simulink model "MainSimLoop"  (R2020b)
settings: Solver=VariableStepAuto  StartTime=0.0  StopTime=30  RelTol=1e-3
values from neighbouring files (symbols this model uses):
  D = 12    [Startup.m]
  dctcq = [-2.56941525e-08,-5.1388305e-08,-2.56941525e-08,2.56941525e-08,5.1388305e-08,2.56941525e-08;     4.45035775874229e-08,0,-4.45035775874229e-08,-4.45035775874229e-08,0,4.45035775874229e-08;     2.925e-09,-2.925e-09,2.925e-09,-2.925e-09,2.925e-09,-2.925e-09]    [Startup.m]
  Jm = 2.9387e-05    [Startup.m]
  mass = 3.3    [Startup.m]
  P = 3.8    [Startup.m]
  X = [ 0, 0, 5, 5, 5, 5, 0]*1    [Path_Construction_Demo_Script.m]
  Y = [ 0, 0, 0, 0, 5, 5, 5]*1    [Path_Construction_Demo_Script.m]
  Z = [ 1, 1, 1, 1, 1, 1, 1]*0    [Path_Construction_Demo_Script.m]
undefined symbols (not defined in the file or in its folder): Newton, Raphson, sigbuilder_block, smiData
libraries: sm_lib x542, fl_lib x73, nesl_utility x26, Electrical_Library x18, pid_lib x12, Mechanical_Library x12, sharedtransform x12, shared6dof x1
(part 4 of 12)

== system MainSimLoop/Quadcopter Dynamics/Motor6CCW/Subsystem ==
  ArmMotorConnector_1_RIGID : Subsystem
  ArmRod_1_RIGID : Subsystem
  LegBodyConnector_1_RIGID : Subsystem
  MotorMount_1_RIGID : Subsystem
  MotorQuad_1_RIGID : Subsystem
  Transform : sm_lib/Frames and Transforms/Rigid Transform  TranslationMethod=Cartesian  TranslationStandardOffset=0  TranslationLengthUnit=mm  TranslationStandardAxis=+Z  TranslationCartesianOffset=smiData.RigidTransform(156).translation  TranslationROffset=0  TranslationROffsetUnits=m  TranslationZOffset=0  TranslationZOffsetUnits=m  TranslationThetaOffset=0  TranslationThetaOffsetUnits=deg  RotationMethod=ArbitraryAxis  RotationAngleUnits=rad  RotationStandardAxis=+Z  RotationAngle=smiData.RigidTransform(156).angle  RotationArbitraryAxis=smiData.RigidTransform(156).axis  FollAlignAxisA=+X  BaseAlignAxisA=+Y  FollAlignAxisB=+Y  BaseAlignAxisB=+Z  RotationSequenceAxes=FollowerAxes  RotationSequence=XYX  RotationSequenceAngles=[0 0 0]  RotationSequenceAnglesUnits=deg  RotationMatrix=[1 0 0; 0 1 0; 0 0 1]
  Transform1 : sm_lib/Frames and Transforms/Rigid Transform  TranslationMethod=Cartesian  TranslationStandardOffset=0  TranslationLengthUnit=mm  TranslationStandardAxis=+Z  TranslationCartesianOffset=smiData.RigidTransform(157).translation  TranslationROffset=0  TranslationROffsetUnits=m  TranslationZOffset=0  TranslationZOffsetUnits=m  TranslationThetaOffset=0  TranslationThetaOffsetUnits=deg  RotationMethod=ArbitraryAxis  RotationAngleUnits=rad  RotationStandardAxis=+Z  RotationAngle=smiData.RigidTransform(157).angle  RotationArbitraryAxis=smiData.RigidTransform(157).axis  FollAlignAxisA=+X  BaseAlignAxisA=+Y  FollAlignAxisB=+Y  BaseAlignAxisB=+Z  RotationSequenceAxes=FollowerAxes  RotationSequence=XYX  RotationSequenceAngles=[0 0 0]  RotationSequenceAnglesUnits=deg  RotationMatrix=[1 0 0; 0 1 0; 0 0 1]
  Transform2 : sm_lib/Frames and Transforms/Rigid Transform  TranslationMethod=Cartesian  TranslationStandardOffset=0  TranslationLengthUnit=mm  TranslationStandardAxis=+Z  TranslationCartesianOffset=smiData.RigidTransform(158).translation  TranslationROffset=0  TranslationROffsetUnits=m  TranslationZOffset=0  TranslationZOffsetUnits=m  TranslationThetaOffset=0  TranslationThetaOffsetUnits=deg  RotationMethod=ArbitraryAxis  RotationAngleUnits=rad  RotationStandardAxis=+Z  RotationAngle=smiData.RigidTransform(158).angle  RotationArbitraryAxis=smiData.RigidTransform(158).axis  FollAlignAxisA=+X  BaseAlignAxisA=+Y  FollAlignAxisB=+Y  BaseAlignAxisB=+Z  RotationSequenceAxes=FollowerAxes  RotationSequence=XYX  RotationSequenceAngles=[0 0 0]  RotationSequenceAnglesUnits=deg  RotationMatrix=[1 0 0; 0 1 0; 0 0 1]
  Transform3 : sm_lib/Frames and Transforms/Rigid Transform  TranslationMethod=Cartesian  TranslationStandardOffset=0  TranslationLengthUnit=mm  TranslationStandardAxis=+Z  TranslationCartesianOffset=smiData.RigidTransform(159).translation  TranslationROffset=0  TranslationROffsetUnits=m  TranslationZOffset=0  TranslationZOffsetUnits=m  TranslationThetaOffset=0  TranslationThetaOffsetUnits=deg  RotationMethod=ArbitraryAxis  RotationAngleUnits=rad  RotationStandardAxis=+Z  RotationAngle=smiData.RigidTransform(159).angle  RotationArbitraryAxis=smiData.RigidTransform(159).axis  FollAlignAxisA=+X  BaseAlignAxisA=+Y  FollAlignAxisB=+Y  BaseAlignAxisB=+Z  RotationSequenceAxes=FollowerAxes  RotationSequence=XYX  RotationSequenceAngles=[0 0 0]  RotationSequenceAnglesUnits=deg  RotationMatrix=[1 0 0; 0 1 0; 0 0 1]
  Transform5 : sm_lib/Frames and Transforms/Rigid Transform  TranslationMethod=Cartesian  TranslationStandardOffset=0  TranslationLengthUnit=mm  TranslationStandardAxis=+Z  TranslationCartesianOffset=smiData.RigidTransform(161).translation  TranslationROffset=0  TranslationROffsetUnits=m  TranslationZOffset=0  TranslationZOffsetUnits=m  TranslationThetaOffset=0  TranslationThetaOffsetUnits=deg  RotationMethod=ArbitraryAxis  RotationAngleUnits=rad  RotationStandardAxis=+Z  RotationAngle=smiData.RigidTransform(161).angle  RotationArbitraryAxis=smiData.RigidTransform(161).axis  FollAlignAxisA=+X  BaseAlignAxisA=+Y  FollAlignAxisB=+Y  BaseAlignAxisB=+Z  RotationSequenceAxes=FollowerAxes  RotationSequence=XYX  RotationSequenceAngles=[0 0 0]  RotationSequenceAnglesUnits=deg  RotationMatrix=[1 0 0; 0 1 0; 0 0 1]
  Transform4 : PMIOPort  Side=Left
  Transform6 : PMIOPort  Port=2  Side=Left
  Transform7 : PMIOPort  Port=3  Side=Left
  connections:
  Transform6/RConn1 -- Transform3/LConn1
  Transform/LConn1 -- Transform1/LConn1 -- Transform2/LConn1 -- Transform7/RConn1
  MotorMount_1_RIGID/LConn1 -- Transform/RConn1
  Transform4/RConn1 -- Transform5/LConn1
  ArmMotorConnector_1_RIGID/LConn1 -- Transform2/RConn1
  MotorQuad_1_RIGID/LConn1 -- Transform5/RConn1
  ArmRod_1_RIGID/LConn1 -- Transform3/RConn1
  LegBodyConnector_1_RIGID/LConn1 -- Transform1/RConn1

== system MainSimLoop/Quadcopter Dynamics/Motor6CCW/xoar_12_4_5CW_1_RIGID ==
  ReferenceFrame : sm_lib/Frames and Transforms/Reference Frame
  Solid : sm_lib/Body Elements/File Solid  ExtGeomFileName=xoar_12_4-5CW_Default_sldprt.STEP  UnitType=FromFile  ExtGeomFileUnits=m  StepReaderType=HEX  ExportConvexHullGeometry=off  InertiaType=Custom  Mass=smiData.Solid(44).mass  MassUnits=kg  CenterOfMass=smiData.Solid(44).CoM  CenterOfMassUnits=m  MomentsOfInertia=smiData.Solid(44).MoI  MomentsOfInertiaUnits=kg*m^2  ProductsOfInertia=smiData.Solid(44).PoI  ProductsOfInertiaUnits=kg*m^2  BasedOnType=DensityFromFile  Density=1000  DensityUnits=kg/m^3  DoExposeReferenceFrame=on  SerializedFrames=<Frames/>  GraphicType=FromGeometry  MarkerShape=Sphere  MarkerSize=10  GraphicVisPropType=SimpleVisualProperties  GraphicDiffuseColor=smiData.Solid(44).color  GraphicSpecularColor=[0.5 0.5 0.5 1.0]  GraphicAmbientColor=[0.15 0.15 0.15 1.0]  GraphicEmissiveColor=[0.0 0.0 0.0 1.0]  GraphicShininess=75  GraphicOpacity=smiData.Solid(44).opacity
  F : PMIOPort  Side=Left
  connections:
  ReferenceFrame/RConn1 -- Solid/RConn1 -- F/RConn1

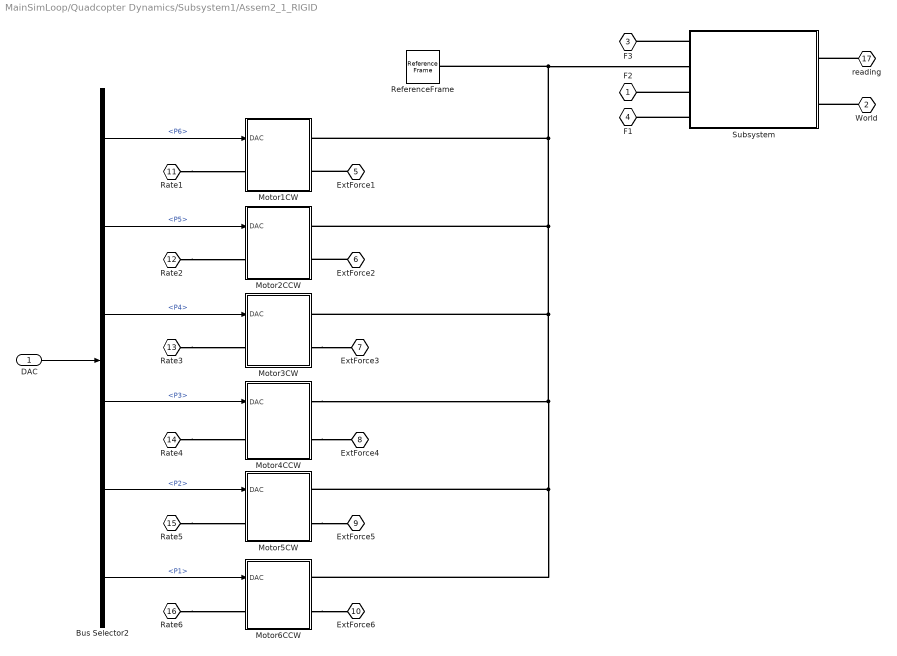
== system MainSimLoop/Quadcopter Dynamics/Subsystem1/Assem2_1_RIGID ==
  DAC : Inport
  Bus Selector2 : BusSelector  OutputSignals=P6,P5,P4,P3,P2,P1
  Motor1CW : Subsystem
  Motor2CCW : Subsystem
  Motor3CW : Subsystem
  Motor4CCW : Subsystem
  Motor5CW : Subsystem
  Motor6CCW : Subsystem
  ReferenceFrame : sm_lib/Frames and Transforms/Reference Frame
  Subsystem : Subsystem
  F2 : PMIOPort  Side=Left
  World : PMIOPort  Tag=PMCPort  Port=2  Side=Left
  F3 : PMIOPort  Port=3  Side=Left
  F1 : PMIOPort  Port=4  Side=Left
  ExtForce1 : PMIOPort  Tag=PMCPort  Port=5  Side=Right
  ExtForce2 : PMIOPort  Tag=PMCPort  Port=6  Side=Right
  ExtForce3 : PMIOPort  Tag=PMCPort  Port=7  Side=Right
  ExtForce4 : PMIOPort  Tag=PMCPort  Port=8  Side=Right
  ExtForce5 : PMIOPort  Tag=PMCPort  Port=9  Side=Right
  ExtForce6 : PMIOPort  Tag=PMCPort  Port=10  Side=Right
  Rate1 : PMIOPort  Tag=PMCPort  Port=11  Side=Right
  Rate2 : PMIOPort  Tag=PMCPort  Port=12  Side=Right
  Rate3 : PMIOPort  Tag=PMCPort  Port=13  Side=Right
  Rate4 : PMIOPort  Tag=PMCPort  Port=14  Side=Right
  Rate5 : PMIOPort  Tag=PMCPort  Port=15  Side=Right
  Rate6 : PMIOPort  Tag=PMCPort  Port=16  Side=Right
  reading : PMIOPort  Tag=PMCPort  Port=17  Side=Right
  wires:
  DAC/1 -> Bus Selector2/1
  Bus Selector2/6 -> Motor6CCW/1(DAC)  "<P1>"
  Bus Selector2/5 -> Motor5CW/1(DAC)  "<P2>"
  Bus Selector2/4 -> Motor4CCW/1(DAC)  "<P3>"
  Bus Selector2/3 -> Motor3CW/1(DAC)  "<P4>"
  Bus Selector2/2 -> Motor2CCW/1(DAC)  "<P5>"
  Bus Selector2/1 -> Motor1CW/1(DAC)  "<P6>"
  connections:
  ExtForce1/RConn1 -- Motor1CW/RConn2
  ExtForce2/RConn1 -- Motor2CCW/RConn2
  Motor3CW/RConn2 -- ExtForce3/RConn1
  Motor4CCW/RConn2 -- ExtForce4/RConn1
  Motor5CW/RConn2 -- ExtForce5/RConn1
  Motor6CCW/RConn2 -- ExtForce6/RConn1
  Rate1/RConn1 -- Motor1CW/LConn1
  Rate2/RConn1 -- Motor2CCW/LConn1
  Rate3/RConn1 -- Motor3CW/LConn1
  Rate4/RConn1 -- Motor4CCW/LConn1
  Rate5/RConn1 -- Motor5CW/LConn1
  Rate6/RConn1 -- Motor6CCW/LConn1
  Motor4CCW/RConn1 -- Motor6CCW/RConn1 -- Motor5CW/RConn1 -- Subsystem/LConn2 -- ReferenceFrame/RConn1 -- Motor1CW/RConn1 -- Motor2CCW/RConn1 -- Motor3CW/RConn1
  Subsystem/LConn1 -- F3/RConn1
  reading/RConn1 -- Subsystem/RConn1
  Subsystem/LConn3 -- F2/RConn1
  Subsystem/LConn4 -- F1/RConn1
  World/RConn1 -- Subsystem/RConn2

== system MainSimLoop/Quadcopter Dynamics/Subsystem1/RotorThrust1 ==
  External Force  and Torque : sm_lib/Forces and Torques/External Force and Torque  ForceResolutionFrame=AttachedFrame  EnableForceX=off  EnableForceY=off  EnableForceZ=on  EnableForce=off  TorqueResolutionFrame=AttachedFrame  EnableTorqueX=off  EnableTorqueY=off  EnableTorqueZ=off  EnableTorque=off
  PS Abs : fl_lib/Physical Signals/Nonlinear Operators/PS Abs
      settings: SourceProductBaseCode=SS  InternalSimscapePortConfiguration="{\"Bottom\":[],\"Left\":[{\"id\":\"I\",\"label\":\"\",\"type\":\"input\"}],\"Right\":[{\"id\":\"O\",\"label\":\"\",\"type\":\"output\"}],\"Top\":[]}"
  PS Constant : fl_lib/Physical Signals/Sources/PS Constant  constant=4.23333e-4*P
  PS Constant1 : fl_lib/Physical Signals/Sources/PS Constant  constant=4.392399e-8*D^3.5/sqrt(P) N
  PS Constant2 : fl_lib/Physical Signals/Sources/PS Constant  constant=1 rad/s
  PS Constant3 : fl_lib/Physical Signals/Sources/PS Constant  constant=1 m/s
  PS Divide : fl_lib/Physical Signals/Functions/PS Divide
      settings: SourceProductBaseCode=SS
  PS Divide1 : fl_lib/Physical Signals/Functions/PS Divide
      settings: SourceProductBaseCode=SS
  PS Gain : fl_lib/Physical Signals/Functions/PS Gain  gain=30/pi
  PS Product : fl_lib/Physical Signals/Functions/PS Product
  PS Product1 : fl_lib/Physical Signals/Functions/PS Product
  PS Product2 : fl_lib/Physical Signals/Functions/PS Product
  PS Subtract : fl_lib/Physical Signals/Functions/PS Subtract
  OmegaProp : PMIOPort  Side=Left
  Thrust : PMIOPort  Port=2  Side=Right
  W : PMIOPort  Port=3  Side=Left
  Reading : PMIOPort  Port=4  Side=Right
  connections:
  External Force  and Torque/RConn1 -- Thrust/RConn1
  PS Product2/RConn1 -- Reading/RConn1 -- External Force  and Torque/LConn1
  PS Gain/LConn1 -- OmegaProp/RConn1
  PS Constant/RConn1 -- PS Product/LConn2
  PS Abs/RConn1 -- PS Product/LConn1 -- PS Product1/LConn1
  PS Product/RConn1 -- PS Subtract/LConn1
  PS Divide1/LConn1 -- W/RConn1
  PS Subtract/RConn1 -- PS Product1/LConn2
  PS Constant1/RConn1 -- PS Product2/LConn2
  PS Product1/RConn1 -- PS Product2/LConn1
  PS Gain/RConn1 -- PS Divide/LConn1
  PS Divide/RConn1 -- PS Abs/LConn1
  PS Constant2/RConn1 -- PS Divide/LConn2
  PS Divide1/RConn1 -- PS Subtract/LConn2
  PS Constant3/RConn1 -- PS Divide1/LConn2

== system MainSimLoop/Quadcopter Dynamics/Subsystem1/RotorThrust2 ==
  External Force  and Torque : sm_lib/Forces and Torques/External Force and Torque  ForceResolutionFrame=AttachedFrame  EnableForceX=off  EnableForceY=off  EnableForceZ=on  EnableForce=off  TorqueResolutionFrame=AttachedFrame  EnableTorqueX=off  EnableTorqueY=off  EnableTorqueZ=off  EnableTorque=off
  PS Abs : fl_lib/Physical Signals/Nonlinear Operators/PS Abs
      settings: SourceProductBaseCode=SS  InternalSimscapePortConfiguration="{\"Bottom\":[],\"Left\":[{\"id\":\"I\",\"label\":\"\",\"type\":\"input\"}],\"Right\":[{\"id\":\"O\",\"label\":\"\",\"type\":\"output\"}],\"Top\":[]}"
  PS Constant : fl_lib/Physical Signals/Sources/PS Constant  constant=4.23333e-4*P
  PS Constant1 : fl_lib/Physical Signals/Sources/PS Constant  constant=4.392399e-8*D^3.5/sqrt(P) N
  PS Constant2 : fl_lib/Physical Signals/Sources/PS Constant  constant=1 rad/s
  PS Constant3 : fl_lib/Physical Signals/Sources/PS Constant  constant=1 m/s
  PS Divide : fl_lib/Physical Signals/Functions/PS Divide
      settings: SourceProductBaseCode=SS
  PS Divide1 : fl_lib/Physical Signals/Functions/PS Divide
      settings: SourceProductBaseCode=SS
  PS Gain : fl_lib/Physical Signals/Functions/PS Gain  gain=30/pi
  PS Product : fl_lib/Physical Signals/Functions/PS Product
  PS Product1 : fl_lib/Physical Signals/Functions/PS Product
  PS Product2 : fl_lib/Physical Signals/Functions/PS Product
  PS Subtract : fl_lib/Physical Signals/Functions/PS Subtract
  OmegaProp : PMIOPort  Side=Left
  Thrust : PMIOPort  Port=2  Side=Right
  W : PMIOPort  Port=3  Side=Left
  Reading : PMIOPort  Port=4  Side=Right
  connections:
  External Force  and Torque/RConn1 -- Thrust/RConn1
  PS Product2/RConn1 -- Reading/RConn1 -- External Force  and Torque/LConn1
  PS Gain/LConn1 -- OmegaProp/RConn1
  PS Constant/RConn1 -- PS Product/LConn2
  PS Abs/RConn1 -- PS Product/LConn1 -- PS Product1/LConn1
  PS Product/RConn1 -- PS Subtract/LConn1
  PS Divide1/LConn1 -- W/RConn1
  PS Subtract/RConn1 -- PS Product1/LConn2
  PS Constant1/RConn1 -- PS Product2/LConn2
  PS Product1/RConn1 -- PS Product2/LConn1
  PS Gain/RConn1 -- PS Divide/LConn1
  PS Divide/RConn1 -- PS Abs/LConn1
  PS Constant2/RConn1 -- PS Divide/LConn2
  PS Divide1/RConn1 -- PS Subtract/LConn2
  PS Constant3/RConn1 -- PS Divide1/LConn2

== system MainSimLoop/Quadcopter Dynamics/Subsystem1/RotorThrust3 ==
  External Force  and Torque : sm_lib/Forces and Torques/External Force and Torque  ForceResolutionFrame=AttachedFrame  EnableForceX=off  EnableForceY=off  EnableForceZ=on  EnableForce=off  TorqueResolutionFrame=AttachedFrame  EnableTorqueX=off  EnableTorqueY=off  EnableTorqueZ=off  EnableTorque=off
  PS Abs : fl_lib/Physical Signals/Nonlinear Operators/PS Abs
      settings: SourceProductBaseCode=SS  InternalSimscapePortConfiguration="{\"Bottom\":[],\"Left\":[{\"id\":\"I\",\"label\":\"\",\"type\":\"input\"}],\"Right\":[{\"id\":\"O\",\"label\":\"\",\"type\":\"output\"}],\"Top\":[]}"
  PS Constant : fl_lib/Physical Signals/Sources/PS Constant  constant=4.23333e-4*P
  PS Constant1 : fl_lib/Physical Signals/Sources/PS Constant  constant=4.392399e-8*D^3.5/sqrt(P) N
  PS Constant2 : fl_lib/Physical Signals/Sources/PS Constant  constant=1 rad/s
  PS Constant3 : fl_lib/Physical Signals/Sources/PS Constant  constant=1 m/s
  PS Divide : fl_lib/Physical Signals/Functions/PS Divide
      settings: SourceProductBaseCode=SS
  PS Divide1 : fl_lib/Physical Signals/Functions/PS Divide
      settings: SourceProductBaseCode=SS
  PS Gain : fl_lib/Physical Signals/Functions/PS Gain  gain=30/pi
  PS Product : fl_lib/Physical Signals/Functions/PS Product
  PS Product1 : fl_lib/Physical Signals/Functions/PS Product
  PS Product2 : fl_lib/Physical Signals/Functions/PS Product
  PS Subtract : fl_lib/Physical Signals/Functions/PS Subtract
  OmegaProp : PMIOPort  Side=Left
  Thrust : PMIOPort  Port=2  Side=Right
  W : PMIOPort  Port=3  Side=Left
  Reading : PMIOPort  Port=4  Side=Right
  connections:
  External Force  and Torque/RConn1 -- Thrust/RConn1
  PS Product2/RConn1 -- Reading/RConn1 -- External Force  and Torque/LConn1
  PS Gain/LConn1 -- OmegaProp/RConn1
  PS Constant/RConn1 -- PS Product/LConn2
  PS Abs/RConn1 -- PS Product/LConn1 -- PS Product1/LConn1
  PS Product/RConn1 -- PS Subtract/LConn1
  PS Divide1/LConn1 -- W/RConn1
  PS Subtract/RConn1 -- PS Product1/LConn2
  PS Constant1/RConn1 -- PS Product2/LConn2
  PS Product1/RConn1 -- PS Product2/LConn1
  PS Gain/RConn1 -- PS Divide/LConn1
  PS Divide/RConn1 -- PS Abs/LConn1
  PS Constant2/RConn1 -- PS Divide/LConn2
  PS Divide1/RConn1 -- PS Subtract/LConn2
  PS Constant3/RConn1 -- PS Divide1/LConn2

== system MainSimLoop/Quadcopter Dynamics/Subsystem1/RotorThrust4 ==
  External Force  and Torque : sm_lib/Forces and Torques/External Force and Torque  ForceResolutionFrame=AttachedFrame  EnableForceX=off  EnableForceY=off  EnableForceZ=on  EnableForce=off  TorqueResolutionFrame=AttachedFrame  EnableTorqueX=off  EnableTorqueY=off  EnableTorqueZ=off  EnableTorque=off
  PS Abs : fl_lib/Physical Signals/Nonlinear Operators/PS Abs
      settings: SourceProductBaseCode=SS  InternalSimscapePortConfiguration="{\"Bottom\":[],\"Left\":[{\"id\":\"I\",\"label\":\"\",\"type\":\"input\"}],\"Right\":[{\"id\":\"O\",\"label\":\"\",\"type\":\"output\"}],\"Top\":[]}"
  PS Constant : fl_lib/Physical Signals/Sources/PS Constant  constant=4.23333e-4*P
  PS Constant1 : fl_lib/Physical Signals/Sources/PS Constant  constant=4.392399e-8*D^3.5/sqrt(P) N
  PS Constant2 : fl_lib/Physical Signals/Sources/PS Constant  constant=1 rad/s
  PS Constant3 : fl_lib/Physical Signals/Sources/PS Constant  constant=1 m/s
  PS Divide : fl_lib/Physical Signals/Functions/PS Divide
      settings: SourceProductBaseCode=SS
  PS Divide1 : fl_lib/Physical Signals/Functions/PS Divide
      settings: SourceProductBaseCode=SS
  PS Gain : fl_lib/Physical Signals/Functions/PS Gain  gain=30/pi
  PS Product : fl_lib/Physical Signals/Functions/PS Product
  PS Product1 : fl_lib/Physical Signals/Functions/PS Product
  PS Product2 : fl_lib/Physical Signals/Functions/PS Product
  PS Subtract : fl_lib/Physical Signals/Functions/PS Subtract
  OmegaProp : PMIOPort  Side=Left
  Thrust : PMIOPort  Port=2  Side=Right
  W : PMIOPort  Port=3  Side=Left
  Reading : PMIOPort  Port=4  Side=Right
  connections:
  External Force  and Torque/RConn1 -- Thrust/RConn1
  PS Product2/RConn1 -- Reading/RConn1 -- External Force  and Torque/LConn1
  PS Gain/LConn1 -- OmegaProp/RConn1
  PS Constant/RConn1 -- PS Product/LConn2
  PS Abs/RConn1 -- PS Product/LConn1 -- PS Product1/LConn1
  PS Product/RConn1 -- PS Subtract/LConn1
  PS Divide1/LConn1 -- W/RConn1
  PS Subtract/RConn1 -- PS Product1/LConn2
  PS Constant1/RConn1 -- PS Product2/LConn2
  PS Product1/RConn1 -- PS Product2/LConn1
  PS Gain/RConn1 -- PS Divide/LConn1
  PS Divide/RConn1 -- PS Abs/LConn1
  PS Constant2/RConn1 -- PS Divide/LConn2
  PS Divide1/RConn1 -- PS Subtract/LConn2
  PS Constant3/RConn1 -- PS Divide1/LConn2

== system MainSimLoop/Quadcopter Dynamics/Subsystem1/RotorThrust5 ==
  External Force  and Torque : sm_lib/Forces and Torques/External Force and Torque  ForceResolutionFrame=AttachedFrame  EnableForceX=off  EnableForceY=off  EnableForceZ=on  EnableForce=off  TorqueResolutionFrame=AttachedFrame  EnableTorqueX=off  EnableTorqueY=off  EnableTorqueZ=off  EnableTorque=off
  PS Abs : fl_lib/Physical Signals/Nonlinear Operators/PS Abs
      settings: SourceProductBaseCode=SS  InternalSimscapePortConfiguration="{\"Bottom\":[],\"Left\":[{\"id\":\"I\",\"label\":\"\",\"type\":\"input\"}],\"Right\":[{\"id\":\"O\",\"label\":\"\",\"type\":\"output\"}],\"Top\":[]}"
  PS Constant : fl_lib/Physical Signals/Sources/PS Constant  constant=4.23333e-4*P
  PS Constant1 : fl_lib/Physical Signals/Sources/PS Constant  constant=4.392399e-8*D^3.5/sqrt(P) N
  PS Constant2 : fl_lib/Physical Signals/Sources/PS Constant  constant=1 rad/s
  PS Constant3 : fl_lib/Physical Signals/Sources/PS Constant  constant=1 m/s
  PS Divide : fl_lib/Physical Signals/Functions/PS Divide
      settings: SourceProductBaseCode=SS
  PS Divide1 : fl_lib/Physical Signals/Functions/PS Divide
      settings: SourceProductBaseCode=SS
  PS Gain : fl_lib/Physical Signals/Functions/PS Gain  gain=30/pi
  PS Product : fl_lib/Physical Signals/Functions/PS Product
  PS Product1 : fl_lib/Physical Signals/Functions/PS Product
  PS Product2 : fl_lib/Physical Signals/Functions/PS Product
  PS Subtract : fl_lib/Physical Signals/Functions/PS Subtract
  OmegaProp : PMIOPort  Side=Left
  Thrust : PMIOPort  Port=2  Side=Right
  W : PMIOPort  Port=3  Side=Left
  Reading : PMIOPort  Port=4  Side=Right
  connections:
  External Force  and Torque/RConn1 -- Thrust/RConn1
  PS Product2/RConn1 -- Reading/RConn1 -- External Force  and Torque/LConn1
  PS Gain/LConn1 -- OmegaProp/RConn1
  PS Constant/RConn1 -- PS Product/LConn2
  PS Abs/RConn1 -- PS Product/LConn1 -- PS Product1/LConn1
  PS Product/RConn1 -- PS Subtract/LConn1
  PS Divide1/LConn1 -- W/RConn1
  PS Subtract/RConn1 -- PS Product1/LConn2
  PS Constant1/RConn1 -- PS Product2/LConn2
  PS Product1/RConn1 -- PS Product2/LConn1
  PS Gain/RConn1 -- PS Divide/LConn1
  PS Divide/RConn1 -- PS Abs/LConn1
  PS Constant2/RConn1 -- PS Divide/LConn2
  PS Divide1/RConn1 -- PS Subtract/LConn2
  PS Constant3/RConn1 -- PS Divide1/LConn2

== system MainSimLoop/Quadcopter Dynamics/Subsystem1/RotorThrust6 ==
  External Force  and Torque : sm_lib/Forces and Torques/External Force and Torque  ForceResolutionFrame=AttachedFrame  EnableForceX=off  EnableForceY=off  EnableForceZ=on  EnableForce=off  TorqueResolutionFrame=AttachedFrame  EnableTorqueX=off  EnableTorqueY=off  EnableTorqueZ=off  EnableTorque=off
  PS Abs : fl_lib/Physical Signals/Nonlinear Operators/PS Abs
      settings: SourceProductBaseCode=SS  InternalSimscapePortConfiguration="{\"Bottom\":[],\"Left\":[{\"id\":\"I\",\"label\":\"\",\"type\":\"input\"}],\"Right\":[{\"id\":\"O\",\"label\":\"\",\"type\":\"output\"}],\"Top\":[]}"
  PS Constant : fl_lib/Physical Signals/Sources/PS Constant  constant=4.23333e-4*P
  PS Constant1 : fl_lib/Physical Signals/Sources/PS Constant  constant=4.392399e-8*D^3.5/sqrt(P) N
  PS Constant2 : fl_lib/Physical Signals/Sources/PS Constant  constant=1 rad/s
  PS Constant3 : fl_lib/Physical Signals/Sources/PS Constant  constant=1 m/s
  PS Divide : fl_lib/Physical Signals/Functions/PS Divide
      settings: SourceProductBaseCode=SS
  PS Divide1 : fl_lib/Physical Signals/Functions/PS Divide
      settings: SourceProductBaseCode=SS
  PS Gain : fl_lib/Physical Signals/Functions/PS Gain  gain=30/pi
  PS Product : fl_lib/Physical Signals/Functions/PS Product
  PS Product1 : fl_lib/Physical Signals/Functions/PS Product
  PS Product2 : fl_lib/Physical Signals/Functions/PS Product
  PS Subtract : fl_lib/Physical Signals/Functions/PS Subtract
  OmegaProp : PMIOPort  Side=Left
  Thrust : PMIOPort  Port=2  Side=Right
  W : PMIOPort  Port=3  Side=Left
  Reading : PMIOPort  Port=4  Side=Right
  connections:
  External Force  and Torque/RConn1 -- Thrust/RConn1
  PS Product2/RConn1 -- Reading/RConn1 -- External Force  and Torque/LConn1
  PS Gain/LConn1 -- OmegaProp/RConn1
  PS Constant/RConn1 -- PS Product/LConn2
  PS Abs/RConn1 -- PS Product/LConn1 -- PS Product1/LConn1
  PS Product/RConn1 -- PS Subtract/LConn1
  PS Divide1/LConn1 -- W/RConn1
  PS Subtract/RConn1 -- PS Product1/LConn2
  PS Constant1/RConn1 -- PS Product2/LConn2
  PS Product1/RConn1 -- PS Product2/LConn1
  PS Gain/RConn1 -- PS Divide/LConn1
  PS Divide/RConn1 -- PS Abs/LConn1
  PS Constant2/RConn1 -- PS Divide/LConn2
  PS Divide1/RConn1 -- PS Subtract/LConn2
  PS Constant3/RConn1 -- PS Divide1/LConn2

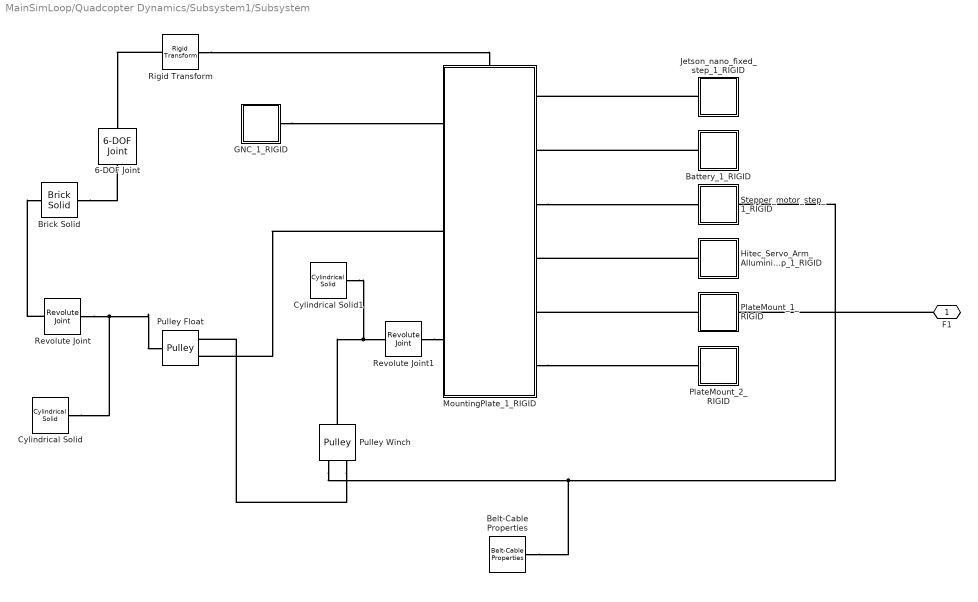
== system MainSimLoop/Quadcopter Dynamics/Subsystem1/Subsystem ==
  6-DOF Joint : sm_lib/Joints/6-DOF Joint  JointMode=Normal  SenseConstraintForce=off  SenseConstraintForceX=off  SenseConstraintForceY=off  SenseConstraintForceZ=off  SenseConstraintTorque=off  SenseConstraintTorqueX=off  SenseConstraintTorqueY=off  SenseConstraintTorqueZ=off  SenseTotalForce=off  SenseTotalForceX=off  SenseTotalForceY=off  SenseTotalForceZ=off  SenseTotalTorque=off  SenseTotalTorqueX=off  SenseTotalTorqueY=off  SenseTotalTorqueZ=off  CompositeWrenchDir=FollowerOnBase  CompositeWrenchFrame=BaseFrame  PxEquilibriumPosition=0  PxEquilibriumPositionUnits=m  PxSpringStiffness=0  PxSpringStiffnessUnits=N/m  PxDampingCoefficient=0  PxDampingCoefficientUnits=N/(m/s)  PxTorqueActuationMode=NoTorque  PxMotionActuationMode=ComputedMotion  PxSensePosition=off  PxSenseVelocity=off  PxSenseAcceleration=off  PxSenseTorqueForce=off  PxSenseLowerLimitTorqueForce=off  PxSenseUpperLimitTorqueForce=off  PxLowerLimitSpecify=off  PxLowerLimitBound=-1  PxLowerLimitBoundUnits=m  PxLowerLimitStiffness=1e6  PxLowerLimitStiffnessUnits=N/m  PxLowerLimitDamping=1e3  PxLowerLimitDampingUnits=N/(m/s)  PxLowerLimitTransitionRegionWidth=1e-4  PxLowerLimitTransitionRegionWidthUnits=m  PxUpperLimitSpecify=off  PxUpperLimitBound=1  PxUpperLimitBoundUnits=m  PxUpperLimitStiffness=1e6  PxUpperLimitStiffnessUnits=N/m  PxUpperLimitDamping=1e3  PxUpperLimitDampingUnits=N/(m/s)  PxUpperLimitTransitionRegionWidth=1e-4  PxUpperLimitTransitionRegionWidthUnits=m  PxPositionTargetSpecify=off  PxPositionTargetPriority=High  PxPositionTargetValue=0  PxPositionTargetValueUnits=m  PxVelocityTargetSpecify=off  PxVelocityTargetPriority=High  PxVelocityTargetValue=0  PxVelocityTargetValueUnits=m/s  PyEquilibriumPosition=0  PyEquilibriumPositionUnits=m  PySpringStiffness=0  PySpringStiffnessUnits=N/m  PyDampingCoefficient=0  PyDampingCoefficientUnits=N/(m/s)  PyTorqueActuationMode=NoTorque  PyMotionActuationMode=ComputedMotion  PySensePosition=off  PySenseVelocity=off  PySenseAcceleration=off  PySenseTorqueForce=off  PySenseLowerLimitTorqueForce=off  PySenseUpperLimitTorqueForce=off  PyLowerLimitSpecify=off  PyLowerLimitBound=-1  PyLowerLimitBoundUnits=m  PyLowerLimitStiffness=1e6  PyLowerLimitStiffnessUnits=N/m  PyLowerLimitDamping=1e3  PyLowerLimitDampingUnits=N/(m/s)  PyLowerLimitTransitionRegionWidth=1e-4  PyLowerLimitTransitionRegionWidthUnits=m  PyUpperLimitSpecify=off  PyUpperLimitBound=1  PyUpperLimitBoundUnits=m  PyUpperLimitStiffness=1e6  PyUpperLimitStiffnessUnits=N/m  PyUpperLimitDamping=1e3  PyUpperLimitDampingUnits=N/(m/s)  PyUpperLimitTransitionRegionWidth=1e-4  PyUpperLimitTransitionRegionWidthUnits=m  PyPositionTargetSpecify=off  PyPositionTargetPriority=High  PyPositionTargetValue=0  PyPositionTargetValueUnits=m  PyVelocityTargetSpecify=off  PyVelocityTargetPriority=High  PyVelocityTargetValue=0  PyVelocityTargetValueUnits=m/s  PzEquilibriumPosition=0  PzEquilibriumPositionUnits=m  PzSpringStiffness=0  PzSpringStiffnessUnits=N/m  PzDampingCoefficient=0  PzDampingCoefficientUnits=N/(m/s)  PzTorqueActuationMode=NoTorque  PzMotionActuationMode=ComputedMotion  PzSensePosition=off  PzSenseVelocity=off  PzSenseAcceleration=off  PzSenseTorqueForce=off  PzSenseLowerLimitTorqueForce=off  PzSenseUpperLimitTorqueForce=off  PzLowerLimitSpecify=off  PzLowerLimitBound=-1  PzLowerLimitBoundUnits=m  PzLowerLimitStiffness=1e6  PzLowerLimitStiffnessUnits=N/m  PzLowerLimitDamping=1e3  PzLowerLimitDampingUnits=N/(m/s)  PzLowerLimitTransitionRegionWidth=1e-4  PzLowerLimitTransitionRegionWidthUnits=m  PzUpperLimitSpecify=off  PzUpperLimitBound=1  PzUpperLimitBoundUnits=m  PzUpperLimitStiffness=1e6  PzUpperLimitStiffnessUnits=N/m  PzUpperLimitDamping=1e3  PzUpperLimitDampingUnits=N/(m/s)  PzUpperLimitTransitionRegionWidth=1e-4  PzUpperLimitTransitionRegionWidthUnits=m  PzPositionTargetSpecify=off  PzPositionTargetPriority=High  PzPositionTargetValue=0  PzPositionTargetValueUnits=m  PzVelocityTargetSpecify=off  PzVelocityTargetPriority=High  PzVelocityTargetValue=0  PzVelocityTargetValueUnits=m/s  SphDefPosRotationMethod=None  SphDefPosRotationAngleUnits=deg  SphDefPosRotationStandardAxis=+Z  SphDefPosRotationAngle=0.0  SphDefPosRotationArbitraryAxis=[0 0 1]  SphDefPosFollAlignAxisA=+X  SphDefPosBaseAlignAxisA=+Y  SphDefPosFollAlignAxisB=+Y  SphDefPosBaseAlignAxisB=+Z  SphDefPosRotationSequenceAxes=FollowerAxes  SphDefPosRotationSequence=XYX  SphDefPosRotationSequenceAngles=[0 0 0]  SphDefPosRotationSequenceAnglesUnits=deg  SphDefPosRotationMatrix=[1 0 0; 0 1 0; 0 0 1]  SphEqPosRotationMethod=None  SphEqPosRotationAngleUnits=deg  SphEqPosRotationStandardAxis=+Z  SphEqPosRotationAngle=0.0  SphEqPosRotationArbitraryAxis=[0 0 1]  SphEqPosFollAlignAxisA=+X  SphEqPosBaseAlignAxisA=+Y  SphEqPosFollAlignAxisB=+Y  SphEqPosBaseAlignAxisB=+Z  SphEqPosRotationSequenceAxes=FollowerAxes  SphEqPosRotationSequence=XYX  SphEqPosRotationSequenceAngles=[0 0 0]  SphEqPosRotationSequenceAnglesUnits=deg  SphEqPosRotationMatrix=[1 0 0; 0 1 0; 0 0 1]  SphSpringStiffness=0  SphSpringStiffnessUnits=N*m/deg  SphDampingCoefficient=0  SphDampingCoefficientUnits=N*m/(deg/s)  SphActuateTorqueX=off  SphActuateTorqueY=off  SphActuateTorqueZ=off  SphActuateTorque=off  SphTorqueActuationMode=NoTorque  SphMotionActuationMode=ComputedMotion  SphActuationFrame=BaseFrame  SphSensePosition=off  SphSenseVelocityX=off  SphSenseVelocityY=off  SphSenseVelocityZ=off  SphSenseVelocity=off  SphSenseAccelerationX=off  SphSenseAccelerationY=off  SphSenseAccelerationZ=off  SphSenseAcceleration=off  SphSenseTorqueX=off  SphSenseTorqueY=off  SphSenseTorqueZ=off  SphSenseTorqueForce=off  SphSenseLowerLimitTorqueMag=off  SphSenseUpperLimitTorqueMag=off  SphSensingFrame=BaseFrame  SphLowerLimitSpecify=off  SphLowerLimitBound=15  SphLowerLimitBoundUnits=deg  SphLowerLimitStiffness=1e4  SphLowerLimitStiffnessUnits=N*m/deg  SphLowerLimitDamping=10  SphLowerLimitDampingUnits=N*m/(deg/s)  SphLowerLimitTransitionRegionWidth=0.1  SphLowerLimitTransitionRegionWidthUnits=deg  SphUpperLimitSpecify=off  SphUpperLimitBound=45  SphUpperLimitBoundUnits=deg  SphUpperLimitStiffness=1e4  SphUpperLimitStiffnessUnits=N*m/deg  SphUpperLimitDamping=10  SphUpperLimitDampingUnits=N*m/(deg/s)  SphUpperLimitTransitionRegionWidth=0.1  SphUpperLimitTransitionRegionWidthUnits=deg  SphPositionTargetRotationMethod=None  SphPositionTargetRotationAngleUnits=deg  SphPositionTargetRotationStandardAxis=+Z  SphPositionTargetRotationAngle=0.0  SphPositionTargetRotationArbitraryAxis=[0 0 1]  SphPositionTargetFollAlignAxisA=+X  SphPositionTargetBaseAlignAxisA=+Y  SphPositionTargetFollAlignAxisB=+Y  SphPositionTargetBaseAlignAxisB=+Z  SphPositionTargetRotationSequenceAxes=FollowerAxes  SphPositionTargetRotationSequence=XYX  SphPositionTargetRotationSequenceAngles=[0 0 0]  SphPositionTargetRotationSequenceAnglesUnits=deg  SphPositionTargetRotationMatrix=[1 0 0; 0 1 0; 0 0 1]  SphPositionTargetSpecify=off  SphPositionTargetPriority=High  SphVelocityTargetValue=[0 0 0]  SphVelocityTargetValueUnits=deg/s  SphVelocityTargetSpecify=off  SphVelocityTargetPriority=High  SphVelocityTargetInFollowerFrame=on
  Battery_1_RIGID : Subsystem
  "Belt-Cable Properties " : sm_lib/Belts and Cables/Belt-Cable Properties  DrumBeltCableAlignment=Unrestricted  GraphicType=PitchLine  GraphicVisPropType=SimpleVisualProperties  GraphicDiffuseColor=[0.9 0.35 0]  GraphicSpecularColor=[0.5 0.5 0.5 1.0]  GraphicAmbientColor=[0.15 0.15 0.15 1.0]  GraphicEmissiveColor=[0.0 0.0 0.0 1.0]  GraphicShininess=75  GraphicOpacity=1
      settings: SourceProductName=Multibody
  Brick Solid : sm_lib/Body Elements/Brick Solid  GraphicAmbientColor=[0.15 0.15 0.15 1.0]  BasedOnType=Density  BrickDimensions=[0.2 0.2 .5]  BrickDimensionUnits=m  CenterOfMass=[0 0 0]  CenterOfMassUnits=m  GraphicDiffuseColor=[0.5 0.5 0.5]  Density=30  DensityUnits=kg/m^3  DoExposeReferenceFrame=on  GraphicEmissiveColor=[0.0 0.0 0.0 1.0]  ExportEntireGeometry=off  SerializedFrames=<Frames><Frame><Id>Frame1</Id><Value><Name>F1</Name><Origin><Source>ReferenceFrame</Source><FeatureName></FeatureName></Origin><PrimaryAxis><DefinedDirection>+Z</DefinedDirection><Source>ReferenceFrame</Source><SourceDirection>+X</SourceDirection><FeatureName></FeatureName></PrimaryAxis><SecondaryAxis><DefinedDirection>+X</DefinedDirection><Source>ReferenceFrame</Source><SourceDirection>+Y</SourceDirection><FeatureName></FeatureName></SecondaryAxis></Value></Frame></Frames>  MarkerShape=Sphere  MarkerSize=10  GraphicType=FromGeometry  InertiaType=CalculateFromGeometry  Mass=1  MassUnits=kg  MomentsOfInertia=[1 1 1]  MomentsOfInertiaUnits=kg*m^2  GraphicOpacity=1.0  ProductsOfInertia=[0 0 0]  ProductsOfInertiaUnits=kg*m^2  GraphicShininess=75  GraphicSpecularColor=[0.5 0.5 0.5 1.0]  GraphicVisPropType=SimpleVisualProperties
  Cylindrical Solid : sm_lib/Body Elements/Cylindrical Solid  GraphicAmbientColor=[0.15 0.15 0.15 1.0]  BasedOnType=Density  CenterOfMass=[0 0 0]  CenterOfMassUnits=m  GraphicDiffuseColor=[0.5 0.5 0.5]  CylinderLength=1  CylinderLengthUnits=mm  CylinderRadius=3  CylinderRadiusUnits=mm  Density=1000  DensityUnits=kg/m^3  DoExposeReferenceFrame=on  GraphicEmissiveColor=[0.0 0.0 0.0 1.0]  ExportEntireGeometry=off  SerializedFrames=<Frames/>  MarkerShape=Sphere  MarkerSize=10  GraphicType=FromGeometry  InertiaType=CalculateFromGeometry  Mass=1  MassUnits=kg  MomentsOfInertia=[1 1 1]  MomentsOfInertiaUnits=kg*m^2  GraphicOpacity=1.0  ProductsOfInertia=[0 0 0]  ProductsOfInertiaUnits=kg*m^2  GraphicShininess=75  GraphicSpecularColor=[0.5 0.5 0.5 1.0]  GraphicVisPropType=SimpleVisualProperties
  Cylindrical Solid1 : sm_lib/Body Elements/Cylindrical Solid  GraphicAmbientColor=[0.15 0.15 0.15 1.0]  BasedOnType=Density  CenterOfMass=[0 0 0]  CenterOfMassUnits=m  GraphicDiffuseColor=[0.5 0.5 0.5]  CylinderLength=1  CylinderLengthUnits=mm  CylinderRadius=3  CylinderRadiusUnits=mm  Density=1000  DensityUnits=kg/m^3  DoExposeReferenceFrame=on  GraphicEmissiveColor=[0.0 0.0 0.0 1.0]  ExportEntireGeometry=off  SerializedFrames=<Frames/>  MarkerShape=Sphere  MarkerSize=10  GraphicType=FromGeometry  InertiaType=CalculateFromGeometry  Mass=1  MassUnits=kg  MomentsOfInertia=[1 1 1]  MomentsOfInertiaUnits=kg*m^2  GraphicOpacity=1.0  ProductsOfInertia=[0 0 0]  ProductsOfInertiaUnits=kg*m^2  GraphicShininess=75  GraphicSpecularColor=[0.5 0.5 0.5 1.0]  GraphicVisPropType=SimpleVisualProperties
  GNC_1_RIGID : Subsystem
  Hitec_Servo_Arm_Alluminium_v2_step_1_RIGID : Subsystem
  Jetson_nano_fixed_step_1_RIGID : Subsystem
  MountingPlate_1_RIGID : Subsystem
      settings: PortSchema="{\"entries\":[{\"content\":{\"sides\":[{\"content\":{\"connectorIds\":[\"LConn1\",\"LConn2\",\"LConn3\"]},\"type\":\"ConnectorPlacement.EquallySpacedRectSide\",\"uuid\":\"37f13b48-7fb0-4005-9ca6-f409b9fa684f\"},{\"content\":{\"connectorIds\":[\"RConn1\",\"RConn2\",\"RConn3\",\"RConn4\",\"RConn5\",\"RConn6\"],\"side\":\"RIGHT\"},\"type\":\"ConnectorPlacement.EquallySpacedRectSide\",\"uuid\":\"2d690845-0e7b-4d66-b1ad-be294b10f5dc\"},{\"content\":{\"connectorIds\":[\"LConn4\"],\"side\":\"TOP\"},\"type\":\"ConnectorPlacement.EquallySpacedRectSide\",\"uuid\":\"d357bba5-f9a5-4696-8bfd-4550ff0913df\"},{\"content\":{\"connectorIds\":[],\"side\":\"HIDDEN\"},\"type\":\"ConnectorPlacement.EquallySpacedRectSide\",\"uuid\":\"eec01532-8cab-450c-b7f0-9df1daf8c0d1\"}]},\"type\":\"ConnectorPlacement.EquallySpacedConnector\",\"uuid\":\"3d1dbf3a-4230-4eb4-a06a-dd0537c33645\"}],\"packageUris\":[\"http://schema.mathworks.com/mf0/Connector/R2020b\"],\"version\":\"1.0\"}"
  PlateMount_1_RIGID : Subsystem
  PlateMount_2_RIGID : Subsystem
  Pulley Float : sm_lib/Belts and Cables/Pulley  PitchRadius=1  PitchRadiusUnits=mm  InitialWrapAngleLowerBound=0.0  InitialWrapAngleLowerBoundUnits=deg  SenseWrapAngle=off  SensePulleyAngleA=off  SensePulleyAngleB=off  SenseFleetAngleA=off  SenseFleetAngleB=off
      settings: SourceProductName=Multibody
  Pulley Winch : sm_lib/Belts and Cables/Pulley  PitchRadius=1  PitchRadiusUnits=mm  InitialWrapAngleLowerBound=0.0  InitialWrapAngleLowerBoundUnits=deg  SenseWrapAngle=off  SensePulleyAngleA=off  SensePulleyAngleB=off  SenseFleetAngleA=off  SenseFleetAngleB=off
      settings: SourceProductName=Multibody
  Revolute Joint : sm_lib/Joints/Revolute Joint  JointMode=Normal  SenseConstraintForce=off  SenseConstraintForceX=off  SenseConstraintForceY=off  SenseConstraintForceZ=off  SenseConstraintTorque=off  SenseConstraintTorqueX=off  SenseConstraintTorqueY=off  SenseConstraintTorqueZ=off  SenseTotalForce=off  SenseTotalForceX=off  SenseTotalForceY=off  SenseTotalForceZ=off  SenseTotalTorque=off  SenseTotalTorqueX=off  SenseTotalTorqueY=off  SenseTotalTorqueZ=off  CompositeWrenchDir=FollowerOnBase  CompositeWrenchFrame=BaseFrame  EquilibriumPosition=0  EquilibriumPositionUnits=deg  SpringStiffness=0  SpringStiffnessUnits=N*m/deg  DampingCoefficient=0  DampingCoefficientUnits=N*m/(deg/s)  TorqueActuationMode=NoTorque  MotionActuationMode=ComputedMotion  SensePosition=off  SenseVelocity=off  SenseAcceleration=off  SenseTorqueForce=off  SenseLowerLimitTorqueForce=off  SenseUpperLimitTorqueForce=off  LowerLimitSpecify=off  LowerLimitBound=-90  LowerLimitBoundUnits=deg  LowerLimitStiffness=1e4  LowerLimitStiffnessUnits=N*m/deg  LowerLimitDamping=10  LowerLimitDampingUnits=N*m/(deg/s)  LowerLimitTransitionRegionWidth=0.1  LowerLimitTransitionRegionWidthUnits=deg  UpperLimitSpecify=off  UpperLimitBound=90  UpperLimitBoundUnits=deg  UpperLimitStiffness=1e4  UpperLimitStiffnessUnits=N*m/deg  UpperLimitDamping=10  UpperLimitDampingUnits=N*m/(deg/s)  UpperLimitTransitionRegionWidth=0.1  UpperLimitTransitionRegionWidthUnits=deg  PositionTargetSpecify=off  PositionTargetPriority=High  PositionTargetValue=0  PositionTargetValueUnits=deg  VelocityTargetSpecify=off  VelocityTargetPriority=High  VelocityTargetValue=0  VelocityTargetValueUnits=deg/s
  Revolute Joint1 : sm_lib/Joints/Revolute Joint  JointMode=Normal  SenseConstraintForce=off  SenseConstraintForceX=off  SenseConstraintForceY=off  SenseConstraintForceZ=off  SenseConstraintTorque=off  SenseConstraintTorqueX=off  SenseConstraintTorqueY=off  SenseConstraintTorqueZ=off  SenseTotalForce=off  SenseTotalForceX=off  SenseTotalForceY=off  SenseTotalForceZ=off  SenseTotalTorque=off  SenseTotalTorqueX=off  SenseTotalTorqueY=off  SenseTotalTorqueZ=off  CompositeWrenchDir=FollowerOnBase  CompositeWrenchFrame=BaseFrame  EquilibriumPosition=0  EquilibriumPositionUnits=deg  SpringStiffness=0  SpringStiffnessUnits=N*m/deg  DampingCoefficient=0  DampingCoefficientUnits=N*m/(deg/s)  TorqueActuationMode=NoTorque  MotionActuationMode=ComputedMotion  SensePosition=off  SenseVelocity=off  SenseAcceleration=off  SenseTorqueForce=off  SenseLowerLimitTorqueForce=off  SenseUpperLimitTorqueForce=off  LowerLimitSpecify=off  LowerLimitBound=-90  LowerLimitBoundUnits=deg  LowerLimitStiffness=1e4  LowerLimitStiffnessUnits=N*m/deg  LowerLimitDamping=10  LowerLimitDampingUnits=N*m/(deg/s)  LowerLimitTransitionRegionWidth=0.1  LowerLimitTransitionRegionWidthUnits=deg  UpperLimitSpecify=off  UpperLimitBound=90  UpperLimitBoundUnits=deg  UpperLimitStiffness=1e4  UpperLimitStiffnessUnits=N*m/deg  UpperLimitDamping=10  UpperLimitDampingUnits=N*m/(deg/s)  UpperLimitTransitionRegionWidth=0.1  UpperLimitTransitionRegionWidthUnits=deg  PositionTargetSpecify=off  PositionTargetPriority=High  PositionTargetValue=0  PositionTargetValueUnits=deg  VelocityTargetSpecify=off  VelocityTargetPriority=High  VelocityTargetValue=0  VelocityTargetValueUnits=deg/s
  Rigid Transform : sm_lib/Frames and Transforms/Rigid Transform  TranslationMethod=StandardAxis  TranslationStandardOffset=3  TranslationLengthUnit=m  TranslationStandardAxis=+Y  TranslationCartesianOffset=[0 0 0]  TranslationROffset=0  TranslationROffsetUnits=m  TranslationZOffset=0  TranslationZOffsetUnits=m  TranslationThetaOffset=0  TranslationThetaOffsetUnits=deg  RotationMethod=StandardAxis  RotationAngleUnits=deg  RotationStandardAxis=+Y  RotationAngle=90  RotationArbitraryAxis=[0 0 1]  FollAlignAxisA=+X  BaseAlignAxisA=+Y  FollAlignAxisB=+Y  BaseAlignAxisB=+Z  RotationSequenceAxes=FollowerAxes  RotationSequence=XYX  RotationSequenceAngles=[0 0 0]  RotationSequenceAnglesUnits=deg  RotationMatrix=[1 0 0; 0 1 0; 0 0 1]
  Stepper_motor_step_1_RIGID : Subsystem
  F1 : PMIOPort  Side=Right
  connections:
  Hitec_Servo_Arm_Alluminium_v2_step_1_RIGID/LConn1 -- MountingPlate_1_RIGID/RConn4
  GNC_1_RIGID/RConn1 -- MountingPlate_1_RIGID/LConn1
  PlateMount_1_RIGID/RConn1 -- MountingPlate_1_RIGID/RConn5
  Jetson_nano_fixed_step_1_RIGID/LConn1 -- MountingPlate_1_RIGID/RConn1
  MountingPlate_1_RIGID/RConn6 -- PlateMount_2_RIGID/RConn1
  F1/RConn1 -- PlateMount_1_RIGID/LConn1
  Battery_1_RIGID/RConn1 -- MountingPlate_1_RIGID/RConn2
  MountingPlate_1_RIGID/RConn3 -- Stepper_motor_step_1_RIGID/LConn1
  Pulley Winch/LConn1 -- Cylindrical Solid1/RConn1 -- Revolute Joint1/RConn1
  Pulley Winch/RConn1 -- "Belt-Cable Properties "/LConn1 -- Stepper_motor_step_1_RIGID/RConn1
  Brick Solid/RConn1 -- 6-DOF Joint/RConn1
  MountingPlate_1_RIGID/LConn2 -- Pulley Float/RConn2
  Rigid Transform/LConn1 -- MountingPlate_1_RIGID/LConn4
  Rigid Transform/RConn1 -- 6-DOF Joint/LConn1
  Pulley Winch/RConn2 -- Pulley Float/RConn1
  Pulley Float/LConn1 -- Revolute Joint/RConn1 -- Cylindrical Solid/RConn1
  Revolute Joint1/LConn1 -- MountingPlate_1_RIGID/LConn3
  Revolute Joint/LConn1 -- Brick Solid/LConn1

== system MainSimLoop/Quadcopter Dynamics/Subsystem1/Subsystem1 ==
  Camera_1_RIGID : Subsystem
  DroneBattery_1_RIGID : Subsystem
  PixhawkHolder_1_RIGID : Subsystem
  Vibration_Plate_Connecter_1_RIGID : Subsystem
      settings: PortSchema="{\"entries\":[{\"content\":{\"sides\":[{\"content\":{\"connectorIds\":[]},\"type\":\"ConnectorPlacement.EquallySpacedRectSide\",\"uuid\":\"69c9cab5-409b-4d4a-a55e-1fc01409eaea\"},{\"content\":{\"connectorIds\":[],\"side\":\"RIGHT\"},\"type\":\"ConnectorPlacement.EquallySpacedRectSide\",\"uuid\":\"4cc28f04-1803-4c37-a960-1b4af29214d3\"},{\"content\":{\"connectorIds\":[\"LConn1\"],\"side\":\"TOP\"},\"type\":\"ConnectorPlacement.EquallySpacedRectSide\",\"uuid\":\"31add5b3-1ad9-4905-851e-ae29a4c4ff04\"},{\"content\":{\"connectorIds\":[\"RConn1\"],\"side\":\"BOTTOM\"},\"type\":\"ConnectorPlacement.EquallySpacedRectSide\",\"uuid\":\"891d80e9-b74a-4238-9ae5-9ce5c4c146cc\"},{\"content\":{\"connectorIds\":[],\"side\":\"HIDDEN\"},\"type\":\"ConnectorPlacement.EquallySpacedRectSide\",\"uuid\":\"696f0baa-0b88-41a8-84bb-4e366948af57\"}]},\"type\":\"ConnectorPlacement.EquallySpacedConnector\",\"uuid\":\"7f367e1b-f8d8-4e03-8f09-23be8362140c\"}],\"packageUris\":[\"http://schema.mathworks.com/mf0/Connector/R2020b\"],\"version\":\"1.0\"}"
  Vibration_Plate_Connecter_2_RIGID : Subsystem
  Vibration_damper_2_RIGID : Subsystem
      settings: PortSchema="{\"entries\":[{\"content\":{\"sides\":[{\"content\":{\"connectorIds\":[\"LConn1\"]},\"type\":\"ConnectorPlacement.EquallySpacedRectSide\",\"uuid\":\"2017626d-f6fd-4442-b786-474c677595b7\"},{\"content\":{\"connectorIds\":[\"RConn1\"],\"side\":\"RIGHT\"},\"type\":\"ConnectorPlacement.EquallySpacedRectSide\",\"uuid\":\"fc00dd39-7902-4b31-b9e6-82bd322f5d90\"},{\"content\":{\"connectorIds\":[],\"side\":\"TOP\"},\"type\":\"ConnectorPlacement.EquallySpacedRectSide\",\"uuid\":\"8c134027-9973-46cd-bf32-7a278f2ca6ab\"},{\"content\":{\"connectorIds\":[\"RConn2\"],\"side\":\"BOTTOM\"},\"type\":\"ConnectorPlacement.EquallySpacedRectSide\",\"uuid\":\"1b85ad09-63e6-401d-bd70-46440c664973\"},{\"content\":{\"connectorIds\":[],\"side\":\"HIDDEN\"},\"type\":\"ConnectorPlacement.EquallySpacedRectSide\",\"uuid\":\"f61684bf-0912-496c-90d8-d1068aee83d5\"}]},\"type\":\"ConnectorPlacement.EquallySpacedConnector\",\"uuid\":\"22f52d31-1d2d-408c-91a9-1614f3022824\"}],\"packageUris\":[\"http://schema.mathworks.com/mf0/Connector/R2020b\"],\"version\":\"1.0\"}"
  F1 : PMIOPort  Side=Right
  F2 : PMIOPort  Port=2  Side=Right
  connections:
  Camera_1_RIGID/RConn1 -- Vibration_damper_2_RIGID/LConn1
  Vibration_Plate_Connecter_2_RIGID/LConn1 -- Vibration_damper_2_RIGID/RConn1
  F1/RConn1 -- Vibration_Plate_Connecter_1_RIGID/RConn1
  DroneBattery_1_RIGID/RConn1 -- PixhawkHolder_1_RIGID/LConn1
  F2/RConn1 -- PixhawkHolder_1_RIGID/RConn1
  Vibration_Plate_Connecter_1_RIGID/LConn1 -- Vibration_damper_2_RIGID/RConn2

== system MainSimLoop/Quadcopter Dynamics/Subsystem1/Subsystem2 ==
  DCM : Inport
  AxisRotDefault : sharedtransform/Direction Cosine Matrix to Rotation Angles/AxisRotDefault  SystemSampleTime=-1  VariantActivationTime=update diagram  Latency=0  AutoFrameSizeCalculation=off
      settings: SourceProductBaseCode=AE,PW,MT,UV,VE,VP
  AxisRotZeroR3 : sharedtransform/Direction Cosine Matrix to Rotation Angles/AxisRotZeroR3  SystemSampleTime=-1  VariantActivationTime=update diagram  Latency=0  AutoFrameSizeCalculation=off
      settings: SourceProductBaseCode=AE,PW,MT,UV,VE,VP
  Get DCM Values : sharedtransform/Direction Cosine Matrix to Rotation Angles/Get DCM Values  SystemSampleTime=-1  VariantActivationTime=update diagram  Latency=0  AutoFrameSizeCalculation=off
      settings: SourceProductBaseCode=AE,PW,MT,UV,VE,VP
  If : If  IfExpression=(u1>=1)|(u1<=-1)
  Merge : Merge
  Selector4 : Selector  InputPortWidth=7  IndexOptions=Index vector (dialog)  Indices=3  OutputSizes=1
  Out1 : Outport
  wires:
  Merge/1 -> Out1/1
  If/1 -> AxisRotZeroR3/Action
  Selector4/1 -> If/1  "r21"
  DCM/1 -> Get DCM Values/1
  Get DCM Values/1 -> Selector4/1, AxisRotZeroR3/1, AxisRotDefault/1
  AxisRotDefault/1 -> Merge/2
  AxisRotZeroR3/1 -> Merge/1
  If/2 -> AxisRotDefault/Action

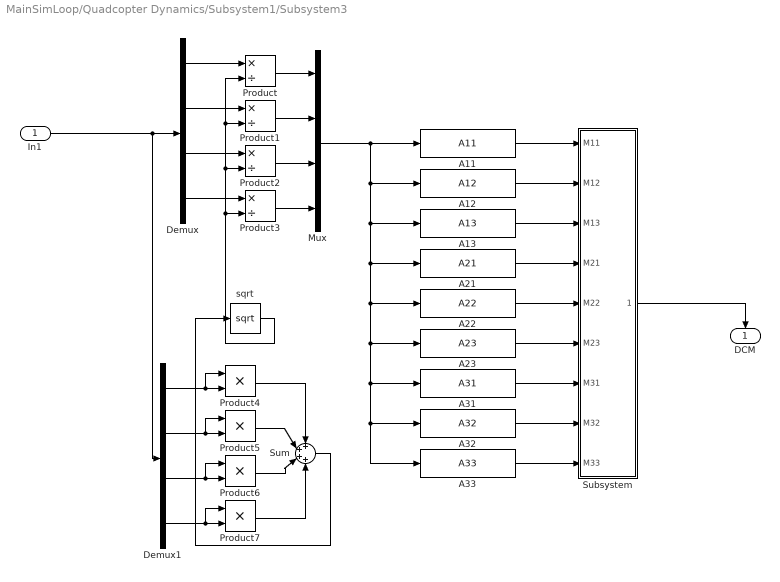
== system MainSimLoop/Quadcopter Dynamics/Subsystem1/Subsystem3 ==
  In1 : Inport
  A11 : sharedtransform/Quaternions to  Direction Cosine Matrix/A11  SystemSampleTime=-1  VariantActivationTime=update diagram  Latency=0  AutoFrameSizeCalculation=off
      settings: SourceProductBaseCode=AE,PW,MT,UV,VE,VP
  A12 : sharedtransform/Quaternions to  Direction Cosine Matrix/A12  SystemSampleTime=-1  VariantActivationTime=update diagram  Latency=0  AutoFrameSizeCalculation=off
      settings: SourceProductBaseCode=AE,PW,MT,UV,VE,VP
  A13 : sharedtransform/Quaternions to  Direction Cosine Matrix/A13  SystemSampleTime=-1  VariantActivationTime=update diagram  Latency=0  AutoFrameSizeCalculation=off
      settings: SourceProductBaseCode=AE,PW,MT,UV,VE,VP
  A21 : sharedtransform/Quaternions to  Direction Cosine Matrix/A21  SystemSampleTime=-1  VariantActivationTime=update diagram  Latency=0  AutoFrameSizeCalculation=off
      settings: SourceProductBaseCode=AE,PW,MT,UV,VE,VP
  A22 : sharedtransform/Quaternions to  Direction Cosine Matrix/A22  SystemSampleTime=-1  VariantActivationTime=update diagram  Latency=0  AutoFrameSizeCalculation=off
      settings: SourceProductBaseCode=AE,PW,MT,UV,VE,VP
  A23 : sharedtransform/Quaternions to  Direction Cosine Matrix/A23  SystemSampleTime=-1  VariantActivationTime=update diagram  Latency=0  AutoFrameSizeCalculation=off
      settings: SourceProductBaseCode=AE,PW,MT,UV,VE,VP
  A31 : sharedtransform/Quaternions to  Direction Cosine Matrix/A31  SystemSampleTime=-1  VariantActivationTime=update diagram  Latency=0  AutoFrameSizeCalculation=off
      settings: SourceProductBaseCode=AE,PW,MT,UV,VE,VP
  A32 : sharedtransform/Quaternions to  Direction Cosine Matrix/A32  SystemSampleTime=-1  VariantActivationTime=update diagram  Latency=0  AutoFrameSizeCalculation=off
      settings: SourceProductBaseCode=AE,PW,MT,UV,VE,VP
  A33 : sharedtransform/Quaternions to  Direction Cosine Matrix/A33  SystemSampleTime=-1  VariantActivationTime=update diagram  Latency=0  AutoFrameSizeCalculation=off
      settings: SourceProductBaseCode=AE,PW,MT,UV,VE,VP
  Demux : Demux
  Demux1 : Demux
  Mux : Mux
  Product{,1..3} (4 alike) : Product  Inputs=*/
  Product{4..7} (4 alike) : Product
  Subsystem : Subsystem
  Sum : Sum  Inputs=4
  sqrt : Sqrt  AlgorithmType=Newton-Raphson  SaturateOnIntegerOverflow=on
  DCM : Outport
  wires:
  Subsystem/1(Matrix) -> DCM/1
  Demux1/4 -> Product7/1, Product7/2
  Demux1/3 -> Product6/1, Product6/2
  A32/1 -> Subsystem/8(M32)
  A31/1 -> Subsystem/7(M31)
  Product5/1 -> Sum/2
  A23/1 -> Subsystem/6(M23)
  A11/1 -> Subsystem/1(M11)
  Product7/1 -> Sum/4
  Mux/1 -> A11/1, A12/1, A13/1, A21/1, A22/1, A23/1, A31/1, A32/1, A33/1
  Sum/1 -> sqrt/1
  A13/1 -> Subsystem/3(M13)
  In1/1 -> Demux1/1, Demux/1
  A21/1 -> Subsystem/4(M21)
  A12/1 -> Subsystem/2(M12)
  A22/1 -> Subsystem/5(M22)
  Demux1/2 -> Product5/1, Product5/2
  Product1/1 -> Mux/2
  A33/1 -> Subsystem/9(M33)
  sqrt/1 -> Product3/2, Product2/2, Product/2, Product1/2
  Product6/1 -> Sum/3
  Product3/1 -> Mux/4
  Demux1/1 -> Product4/1, Product4/2
  Product2/1 -> Mux/3
  Product4/1 -> Sum/1
  Demux/4 -> Product3/1
  Demux/3 -> Product2/1
  Demux/2 -> Product1/1
  Product/1 -> Mux/1
  Demux/1 -> Product/1

== system MainSimLoop/Quadcopter Dynamics/Motor1CW/Subsystem/ArmMotorConnector_1_RIGID ==
  ReferenceFrame : sm_lib/Frames and Transforms/Reference Frame
  Solid : sm_lib/Body Elements/File Solid  ExtGeomFileName=ArmMotorConnector_Default_sldprt.STEP  UnitType=FromFile  ExtGeomFileUnits=m  StepReaderType=HEX  ExportConvexHullGeometry=off  InertiaType=Custom  Mass=smiData.Solid(42).mass  MassUnits=kg  CenterOfMass=smiData.Solid(42).CoM  CenterOfMassUnits=mm  MomentsOfInertia=smiData.Solid(42).MoI  MomentsOfInertiaUnits=kg*mm^2  ProductsOfInertia=smiData.Solid(42).PoI  ProductsOfInertiaUnits=kg*mm^2  BasedOnType=DensityFromFile  Density=1000  DensityUnits=kg/m^3  DoExposeReferenceFrame=on  SerializedFrames=<Frames/>  GraphicType=FromGeometry  MarkerShape=Sphere  MarkerSize=10  GraphicVisPropType=SimpleVisualProperties  GraphicDiffuseColor=smiData.Solid(42).color  GraphicSpecularColor=[0.5 0.5 0.5 1.0]  GraphicAmbientColor=[0.15 0.15 0.15 1.0]  GraphicEmissiveColor=[0.0 0.0 0.0 1.0]  GraphicShininess=75  GraphicOpacity=smiData.Solid(42).opacity
  F : PMIOPort  Side=Left
  connections:
  ReferenceFrame/RConn1 -- Solid/RConn1 -- F/RConn1
